simulink model "cps_base_processor_v2"  (R2012b)
settings: Solver=FixedStepDiscrete  StartTime=0.0  StopTime=8.5  FixedStep=0.005  RelTol=20e-5
model workspace (MAT data in the model file):
  vel_effective_zero = 0.0001
  pos_precision = 0.0006
  board_vpos = 0
  block_height = 0.07
libraries: simulink x4, cps_lib_v2 x3
settings Model: Creator=pmosterm  LastModifiedBy=pmosterm
settings SolverCC: ZcThreshold=2e-5  MaxConsecutiveZCs=20  EnableConcurrentExecution=on  ConcurrentTasks=on  ZeroCrossAlgorithm=Adaptive  SolverResetMethod=Robust
settings DataIOCC: SignalLoggingSaveFormat=ModelDataLogs
settings OptimizationCC: InlineParams=on  ZeroExternalMemoryAtStartup=off  ZeroInternalMemoryAtStartup=off  OptimizeModelRefInitCode=on
settings DebuggingCC: AlgebraicLoopMsg=error  UnderspecifiedInitializationDetection=Simplified  FcnCallInpInsideContextMsg=EnableAllAsWarning  BusObjectLabelMismatch=error  ModelReferenceExtraNoncontSigs=warning
settings ModelReferenceCC: ModelReferenceNumInstancesAllowed=Single
settings RTWCC: SystemTargetFile=autosar.tlc  GenCodeOnly=on  TemplateMakefile=ert_default_tmf  Description=AUTOSAR  ProcessScript=autosar_make_rtw_hook
settings CodeAppCC: IgnoreCustomStorageClasses=off
settings STFCustomTargetCC: CodeReplacementLibrary=ANSI_C  ParMdlRefBuildCompliant=on  CompOptLevelCompliant=on  IncludeMdlTerminateFcn=off  CombineOutputUpdateFcns=on  SuppressErrorStatus=on  ERTFirstTimeCompliant=on  ERTCustomFileBanners=on  SupportNonFinite=off  SupportComplex=off  SupportContinuousTime=off  SupportNonInlinedSFcns=off  AutosarCompliant=on  GRTInterface=off  SystemTargetFile=autosar.tlc
settings ERTTargetCC: CodeReplacementLibrary=ANSI_C  MultiwordLength=2048  ConcurrentExecutionCompliant=off  IncludeMdlTerminateFcn=off  SuppressErrorStatus=on  SupportNonFinite=off  SupportComplex=off  ModelStepFunctionPrototypeControlCompliant=off  CPPClassGenCompliant=off  AutosarCompliant=on  InlinedParameterPlacement=NonHierarchical  ERTCustomFileTemplate=example_file_process.tlc  ConvertIfToSwitch=off  SuppressUnreachableDefaultCases=off
settings ConfigurationSet: Description=SimMechanics 2G

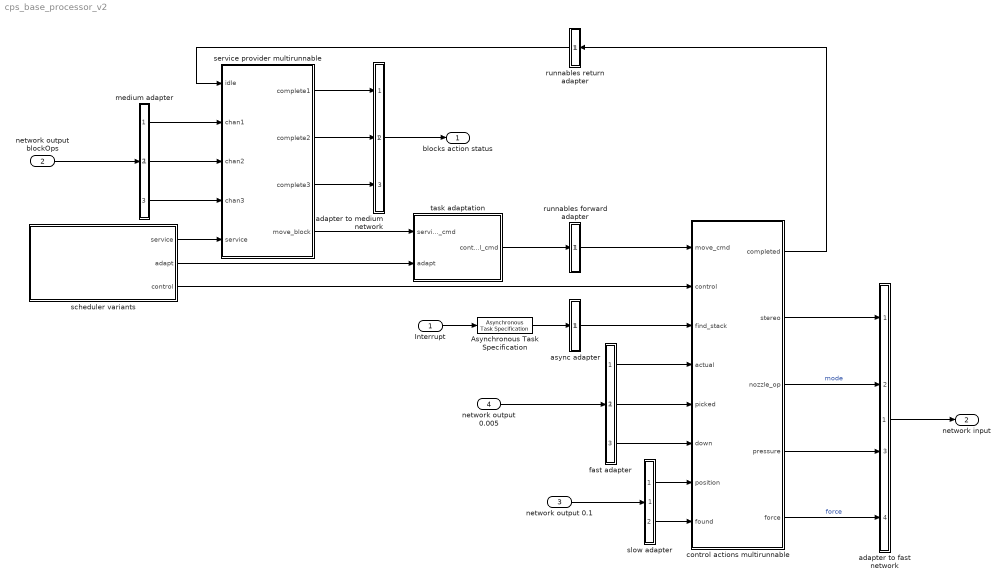
== system cps_base_processor_v2 ==
  Interrupt : Inport  OutputFunctionCall=on
  network output blockOps : Inport  Port=2  OutDataTypeStr=Bus: slBusBlockOps  PortDimensions=3  SampleTime=0.05  BusOutputAsStruct=on
  network output 0.1 : Inport  Port=3  OutDataTypeStr=Bus: slBusStereoOps  SampleTime=0.1  BusOutputAsStruct=on
  network output 0.005 : Inport  Port=4  OutDataTypeStr=Bus: slBusSliderStatus  BusOutputAsStruct=on
  Asynchronous Task Specification : AsynchronousTaskSpecification
  adapter to fast network : Subsystem
      mask Display:
      | patch([0 10 10 0], [0 0 12 0], [1 1 1]);
      | patch([0 10 0 0], [0 12 12 0], [0 0 0]);
      | 
      | plot([0 10 10 0 0], [0 0 12 12 0]);
  adapter to medium network : Subsystem
      mask Display:
      | patch([0 10 10 0], [0 0 12 0], [1 1 1]);
      | patch([0 10 0 0], [0 12 12 0], [0 0 0]);
      | 
      | plot([0 10 10 0 0], [0 0 12 12 0]);
  async adapter : Subsystem
      mask Display:
      | patch([0 10 10 0], [0 0 12 0], [0 0 0]);
      | patch([0 10 0 0], [0 12 12 0], [1 1 1]);
      | 
      | plot([0 10 10 0 0], [0 0 12 12 0]);
  control actions multirunnable : Subsystem
      mask Display:
      | patch([0 13 13 0], [0 0 11 11], [1 1 1]);
      | 
      | patch([1 7 13 1], [0 5 0 0], [0 0 0]);
      | patch([1 7 13 1], [11 6 11 11], [0 0 0]);
      | 
      | plot([7 7], [0 11]);
      | plot([0 13 13 0], [0 0 12 12]);
      | 
      | patch([14 41 41 14 14], [0 0 12 12 0], [1 1 1]);
      | plot([13 42 42 13 13], [0 0 12 12 0]);
      | 
      | text(17,6,'run()');
  fast adapter : Subsystem
      mask Display:
      | patch([0 10 10 0], [0 0 12 0], [0 0 0]);
      | patch([0 10 0 0], [0 12 12 0], [1 1 1]);
      | 
      | plot([0 10 10 0 0], [0 0 12 12 0]);
  medium adapter : Subsystem
      mask Display:
      | patch([0 10 10 0], [0 0 12 0], [0 0 0]);
      | patch([0 10 0 0], [0 12 12 0], [1 1 1]);
      | 
      | plot([0 10 10 0 0], [0 0 12 12 0]);
  runnables forward adapter : Subsystem
      mask Display:
      | patch([0 10 10 0 0], [0 0 10 10 0], [1 1 1]);
      | 
      | patch([0 5 5 0 0], [0 0 4 4 0], [0 0 0]);
      | patch([5 9 9 5 5], [5 5 9 9 5], [0 0 0]);
      | 
      | plot([0 10 10 0 0], [0 0 10 10 0]);
  runnables return adapter : Subsystem
      mask Display:
      | patch([0 10 10 0 0], [0 0 10 10 0], [1 1 1]);
      | 
      | patch([0 5 5 0 0], [0 0 4 4 0], [0 0 0]);
      | patch([5 9 9 5 5], [5 5 9 9 5], [0 0 0]);
      | 
      | plot([0 10 10 0 0], [0 0 10 10 0]);
  scheduler variants : Subsystem  Variant=on
  service provider multirunnable : Subsystem
      mask Display:
      | patch([0 13 13 0], [0 0 11 11], [1 1 1]);
      | 
      | patch([1 7 13 1], [0 5 0 0], [0 0 0]);
      | patch([1 7 13 1], [11 6 11 11], [0 0 0]);
      | 
      | plot([7 7], [0 11]);
      | plot([0 13 13 0], [0 0 12 12]);
      | 
      | patch([14 41 41 14 14], [0 0 12 12 0], [1 1 1]);
      | plot([13 42 42 13 13], [0 0 12 12 0]);
      | 
      | text(17,6,'run()');
  slow adapter : Subsystem
      mask Display:
      | patch([0 10 10 0], [0 0 12 0], [0 0 0]);
      | patch([0 10 0 0], [0 12 12 0], [1 1 1]);
      | 
      | plot([0 10 10 0 0], [0 0 12 12 0]);
  task adaptation : Subsystem
      mask Display:
      | patch([0 13 13 0], [0 0 11 11], [1 1 1]);
      | 
      | patch([1 7 13 1], [0 5 0 0], [0 0 0]);
      | patch([1 7 13 1], [11 6 11 11], [0 0 0]);
      | 
      | plot([7 7], [0 11]);
      | plot([0 13 13 0], [0 0 12 12]);
      | 
      | patch([14 41 41 14 14], [0 0 12 12 0], [1 1 1]);
      | plot([13 42 42 13 13], [0 0 12 12 0]);
      | 
      | text(17,6,'run()');
  blocks action status : Outport  SampleTime=0.05  BusOutputAsStruct=on
  network input : Outport  Port=2  OutDataTypeStr=Bus: slBusBaseOps  SampleTime=0.005  BusOutputAsStruct=on
  wires:
  scheduler variants/1(service) -> service provider multirunnable/5(service)
  scheduler variants/3(control) -> control actions multirunnable/2(control)
  network output blockOps/1 -> medium adapter/1(ops)
  medium adapter/1(R) -> service provider multirunnable/2(chan1)
  medium adapter/2(G) -> service provider multirunnable/3(chan2)
  network output 0.005/1 -> fast adapter/1(In1)
  fast adapter/1(Out1) -> control actions multirunnable/4(actual)
  fast adapter/2(Out2) -> control actions multirunnable/5(picked)
  fast adapter/3(Out3) -> control actions multirunnable/6(down)
  network output 0.1/1 -> slow adapter/1(In1)
  slow adapter/1(Out1) -> control actions multirunnable/7(position)
  slow adapter/2(Out2) -> control actions multirunnable/8(found)
  service provider multirunnable/1(complete1) -> adapter to medium network/1(R)
  service provider multirunnable/2(complete2) -> adapter to medium network/2(G)
  adapter to medium network/1(status) -> blocks action status/1
  control actions multirunnable/2(stereo) -> adapter to fast network/1(In1)
  control actions multirunnable/3(nozzle_op) -> adapter to fast network/2(In2)  "mode"
  control actions multirunnable/4(pressure) -> adapter to fast network/3(In3)
  control actions multirunnable/5(force) -> adapter to fast network/4(In4)  "force"
  adapter to fast network/1(Out1) -> network input/1
  Interrupt/1 -> Asynchronous Task Specification/1
  async adapter/1(find stack) -> control actions multirunnable/3(find_stack)
  Asynchronous Task Specification/1 -> async adapter/1(start operation)
  medium adapter/3(B) -> service provider multirunnable/4(chan3)
  service provider multirunnable/3(complete3) -> adapter to medium network/3(B)
  scheduler variants/2(adapt) -> task adaptation/2(adapt)
  service provider multirunnable/4(move_block) -> task adaptation/1(service_cmd)
  control actions multirunnable/1(completed) -> runnables return adapter/1(In1)
  runnables return adapter/1(Out1) -> service provider multirunnable/1(idle)
  task adaptation/1(control_cmd) -> runnables forward adapter/1(In1)
  runnables forward adapter/1(Out1) -> control actions multirunnable/1(move_cmd)

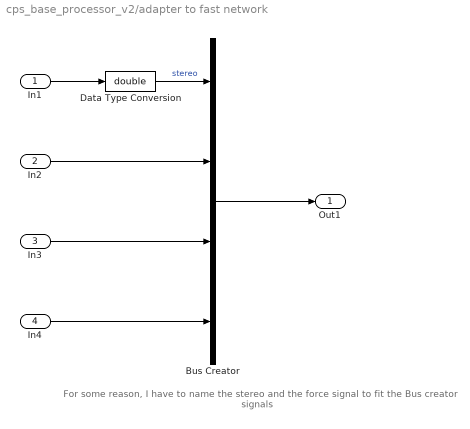
== system cps_base_processor_v2/adapter to fast network ==
  note: For some reason, I have to name
      | the stereo and the force signal
      | to fit the Bus creator signals
  In1 : Inport
  In2 : Inport  Port=2
  In3 : Inport  Port=3
  In4 : Inport  Port=4
  Bus Creator : BusCreator  Inputs='stereo','mode','pressure','force'  OutDataTypeStr=Bus: slBusBaseOps  NonVirtualBus=on
  Data Type Conversion : DataTypeConversion  OutDataTypeStr=double
  Out1 : Outport
  wires:
  Bus Creator/1 -> Out1/1
  In1/1 -> Data Type Conversion/1
  In3/1 -> Bus Creator/3
  In4/1 -> Bus Creator/4
  Data Type Conversion/1 -> Bus Creator/1  "stereo"
  In2/1 -> Bus Creator/2

== system cps_base_processor_v2/adapter to medium network ==
  R : Inport
  G : Inport  Port=2
  B : Inport  Port=3
  Mux1 : Mux  Inputs=3
  Rate Transition4 : RateTransition  Integrity=off  Deterministic=off
  status : Outport
  wires:
  Rate Transition4/1 -> status/1
  Mux1/1 -> Rate Transition4/1
  R/1 -> Mux1/1
  G/1 -> Mux1/2
  B/1 -> Mux1/3

== system cps_base_processor_v2/async adapter ==
  start operation : Inport
  Rate Transition4 : RateTransition  Integrity=off  Deterministic=off
  start finding stack : Subsystem  TreatAsAtomicUnit=on
  find stack : Outport
  wires:
  start operation/1 -> start finding stack/Trigger
  start finding stack/1(find_stack) -> Rate Transition4/1
  Rate Transition4/1 -> find stack/1

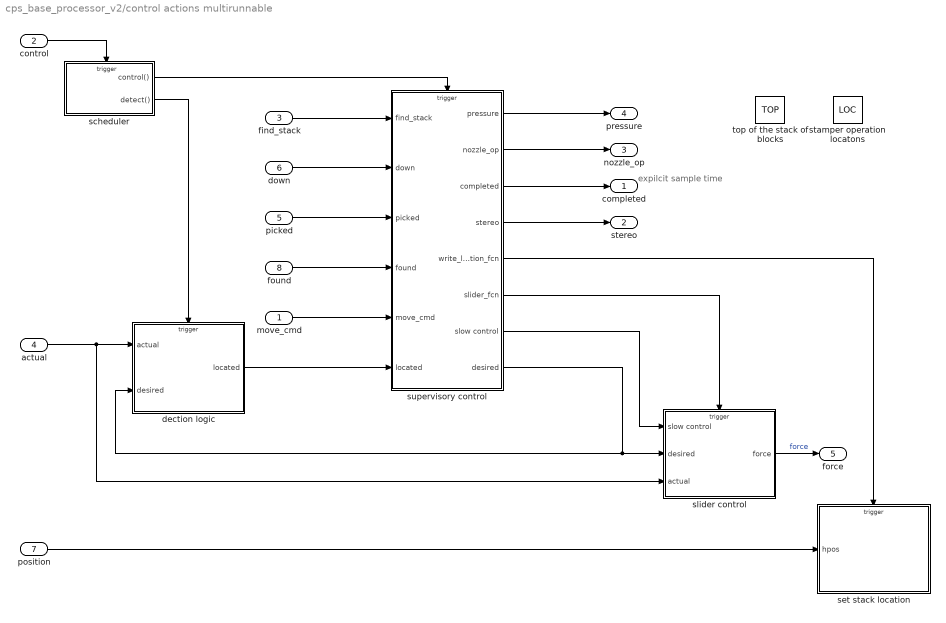
== system cps_base_processor_v2/control actions multirunnable ==
  note: expilcit sample
      | time
  move_cmd : Inport
  control : Inport  Port=2
  find_stack : Inport  Port=3
  actual : Inport  Port=4
  picked : Inport  Port=5
  down : Inport  Port=6
  position : Inport  Port=7
  found : Inport  Port=8
  dection logic : Subsystem
  scheduler : Stateflow chart  TreatAsAtomicUnit=on
  set stack location : Subsystem  TreatAsAtomicUnit=on
  slider control : Subsystem
  stamper operation locatons : DataStoreMemory  DataStoreName=LOC  WriteAfterWriteMsg=warning  InitialValue=[0.4 0.3 -0.05 -0.4 -0.6]  OutDataTypeStr=double
  supervisory control : Subsystem
  top of the stack of blocks : DataStoreMemory  DataStoreName=TOP  WriteAfterWriteMsg=warning  InitialValue=[0 0 0 3 0]  OutDataTypeStr=double
  completed : Outport
  stereo : Outport  Port=2
  nozzle_op : Outport  Port=3
  pressure : Outport  Port=4
  force : Outport  Port=5
  wires:
  position/1 -> set stack location/1(hpos)
  actual/1 -> dection logic/1(actual), slider control/3(actual)
  slider control/1(force) -> force/1  "force"
  find_stack/1 -> supervisory control/1(find_stack)
  down/1 -> supervisory control/2(down)
  picked/1 -> supervisory control/3(picked)
  found/1 -> supervisory control/4(found)
  move_cmd/1 -> supervisory control/5(move_cmd)
  dection logic/1(located) -> supervisory control/6(located)
  supervisory control/1(pressure) -> pressure/1
  supervisory control/2(nozzle_op) -> nozzle_op/1
  supervisory control/3(completed) -> completed/1
  supervisory control/6(slider_fcn) -> slider control/Trigger
  supervisory control/5(write_location_fcn) -> set stack location/Trigger
  scheduler/1(control()) -> supervisory control/Trigger
  scheduler/2(detect()) -> dection logic/Trigger
  supervisory control/4(stereo) -> stereo/1
  supervisory control/7(slow control) -> slider control/1(slow control)
  supervisory control/8(desired) -> slider control/2(desired), dection logic/2(desired)
  control/1 -> scheduler/Trigger

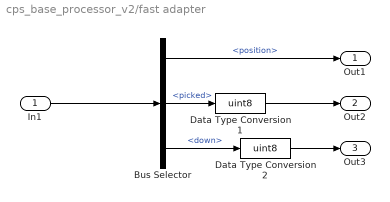
== system cps_base_processor_v2/fast adapter ==
  In1 : Inport
  Bus Selector : BusSelector  OutputSignals=position,picked,down
  Data Type Conversion1 : DataTypeConversion  OutDataTypeStr=uint8
  Data Type Conversion2 : DataTypeConversion  OutDataTypeStr=uint8
  Out1 : Outport
  Out2 : Outport  Port=2
  Out3 : Outport  Port=3
  wires:
  In1/1 -> Bus Selector/1
  Bus Selector/1 -> Out1/1  "<position>"
  Bus Selector/2 -> Data Type Conversion1/1  "<picked>"
  Bus Selector/3 -> Data Type Conversion2/1  "<down>"
  Data Type Conversion1/1 -> Out2/1
  Data Type Conversion2/1 -> Out3/1

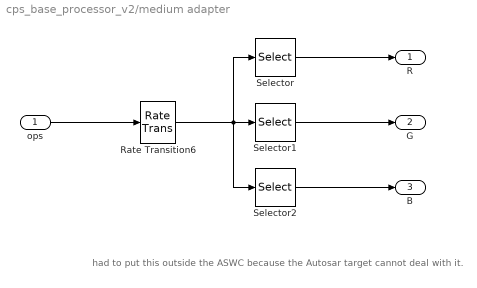
== system cps_base_processor_v2/medium adapter ==
  note: had to put this outside the ASWC
      | because the Autosar target
      | cannot deal with it.
  ops : Inport
  Rate Transition6 : RateTransition  Integrity=off  Deterministic=off
  Selector : Selector  InputPortWidth=3  IndexOptions=Index vector (dialog)  Indices=1  OutputSizes=1
  Selector1 : Selector  InputPortWidth=3  IndexOptions=Index vector (dialog)  Indices=2  OutputSizes=1
  Selector2 : Selector  InputPortWidth=3  IndexOptions=Index vector (dialog)  Indices=3  OutputSizes=1
  R : Outport
  G : Outport  Port=2
  B : Outport  Port=3
  wires:
  ops/1 -> Rate Transition6/1
  Rate Transition6/1 -> Selector2/1, Selector/1, Selector1/1
  Selector/1 -> R/1
  Selector1/1 -> G/1
  Selector2/1 -> B/1

== system cps_base_processor_v2/runnables forward adapter ==
  note: to break dependencies
      | for Autosar target
  In1 : Inport
  Rate Transition3 : RateTransition  Integrity=off  Deterministic=off
  Unit Delay : UnitDelay  SampleTime=-1
  Out1 : Outport
  wires:
  Rate Transition3/1 -> Out1/1
  In1/1 -> Unit Delay/1
  Unit Delay/1 -> Rate Transition3/1

== system cps_base_processor_v2/runnables return adapter ==
  note: to break dependencies
      | for Autosar target
      | otherwise this is only
      | necessary for the multirate
      | scheduler variant
  In1 : Inport
  Rate Transition1 : RateTransition  Integrity=off  Deterministic=off
  Unit Delay : UnitDelay  SampleTime=-1
  Out1 : Outport
  wires:
  Rate Transition1/1 -> Out1/1
  In1/1 -> Unit Delay/1
  Unit Delay/1 -> Rate Transition1/1

== system cps_base_processor_v2/scheduler variants ==
  note: 1) Only subsystems can be added as variant choices at this level
      | 2) Blocks cannot be connected at this level as connectivity is
      | automatically determined at simulation, based on the active variant
  multi rate scheduling : Subsystem  VariantObject=useMultirateVariant
  single rate conditional schaduler : Subsystem  VariantObject=noMultirateVariant
  service : Outport
  adapt : Outport  Port=2
  control : Outport  Port=3

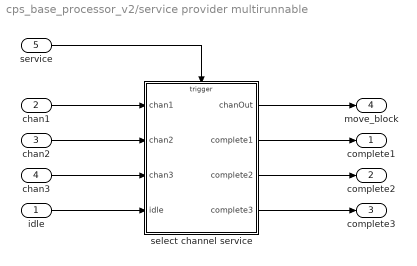
== system cps_base_processor_v2/service provider multirunnable ==
  idle : Inport
  chan1 : Inport  Port=2
  chan2 : Inport  Port=3
  chan3 : Inport  Port=4
  service : Inport  Port=5
  select channel service : Stateflow chart  TreatAsAtomicUnit=on
  complete1 : Outport
  complete2 : Outport  Port=2
  complete3 : Outport  Port=3
  move_block : Outport  Port=4
  wires:
  idle/1 -> select channel service/4(idle)
  select channel service/2(complete1) -> complete1/1
  select channel service/1(chanOut) -> move_block/1
  select channel service/3(complete2) -> complete2/1
  chan1/1 -> select channel service/1(chan1)
  chan2/1 -> select channel service/2(chan2)
  chan3/1 -> select channel service/3(chan3)
  select channel service/4(complete3) -> complete3/1
  service/1 -> select channel service/Trigger

== system cps_base_processor_v2/slow adapter ==
  In1 : Inport
  Bus Selector1 : BusSelector  OutputSignals=location,found
  Data Type Conversion3 : DataTypeConversion  OutDataTypeStr=uint16
  Rate Transition3 : RateTransition  Integrity=off  Deterministic=off
  Out1 : Outport
  Out2 : Outport  Port=2
  wires:
  In1/1 -> Rate Transition3/1
  Rate Transition3/1 -> Bus Selector1/1
  Bus Selector1/1 -> Out1/1  "<location>"
  Bus Selector1/2 -> Data Type Conversion3/1  "<found>"
  Data Type Conversion3/1 -> Out2/1

== system cps_base_processor_v2/task adaptation ==
  service_cmd : Inport
  adapt : Inport  Port=2
  location index offset : Subsystem
  control_cmd : Outport
  wires:
  service_cmd/1 -> location index offset/1(service_cmd)
  adapt/1 -> location index offset/Trigger
  location index offset/1(control_cmd) -> control_cmd/1

== system cps_base_processor_v2/async adapter/start finding stack ==
  fcn : TriggerPort  TriggerType=function-call  PortDimensions=1
  constant : Constant  SampleTime=-1
  find_stack : Outport  OutDataTypeStr=double  PortDimensions=1  OutputWhenDisabled=reset  InitialOutput=0
  wires:
  constant/1 -> find_stack/1

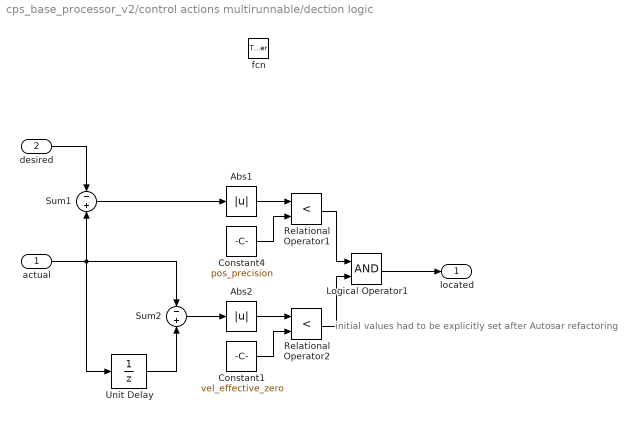
== system cps_base_processor_v2/control actions multirunnable/dection logic ==
  note: initial values had to be explicitly set
      | after Autosar refactoring
  actual : Inport
  desired : Inport  Port=2
  fcn : TriggerPort  TriggerType=function-call  PortDimensions=1
  Abs1 : Abs  ZeroCross=off
  Abs2 : Abs  ZeroCross=off
  Constant1 : Constant  Value=vel_effective_zero  OutDataTypeStr=double
  Constant4 : Constant  Value=pos_precision  OutDataTypeStr=double
  Logical Operator1 : Logic  AllPortsSameDT=off  OutDataTypeStr=boolean
  Relational Operator1 : RelationalOperator  Operator=<  OutDataTypeStr=boolean  ZeroCross=off
  Relational Operator2 : RelationalOperator  Operator=<  OutDataTypeStr=boolean  ZeroCross=off
  Sum1 : Sum  Inputs=-|+
  Sum2 : Sum  Inputs=-|+
  Unit Delay : UnitDelay  SampleTime=-1
  located : Outport  OutDataTypeStr=boolean  PortDimensions=1  InitialOutput=0
  wires:
  Constant4/1 -> Relational Operator1/2
  Sum1/1 -> Abs1/1
  Abs1/1 -> Relational Operator1/1
  actual/1 -> Sum2/1, Unit Delay/1, Sum1/2
  Relational Operator1/1 -> Logical Operator1/1
  Relational Operator2/1 -> Logical Operator1/2
  desired/1 -> Sum1/1
  Abs2/1 -> Relational Operator2/1
  Sum2/1 -> Abs2/1
  Constant1/1 -> Relational Operator2/2
  Unit Delay/1 -> Sum2/2
  Logical Operator1/1 -> located/1

== system cps_base_processor_v2/control actions multirunnable/set stack location ==
  hpos : Inport
  fcn : TriggerPort  TriggerType=function-call
  Demux : Demux  Outputs=5
  LOC = [min pos1 pos2 pos3 max] : DataStoreRead  DataStoreName=LOC
  Mux : Mux  Inputs=5
  Terminator : Terminator
  stamper locations : DataStoreWrite  DataStoreName=LOC
  wires:
  LOC = [min pos1 pos2 pos3 max]/1 -> Demux/1
  Demux/2 -> Mux/2
  Demux/3 -> Mux/3
  Demux/4 -> Terminator/1
  Demux/5 -> Mux/5
  Mux/1 -> stamper locations/1
  hpos/1 -> Mux/4
  Demux/1 -> Mux/1

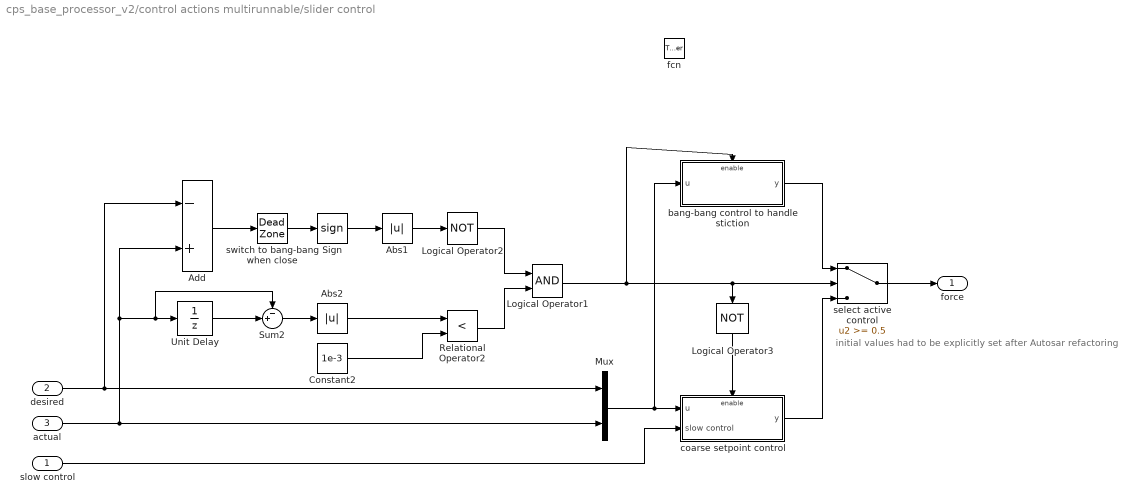
== system cps_base_processor_v2/control actions multirunnable/slider control ==
  note: initial values had to be explicitly set
      | after Autosar refactoring
  slow control : Inport  OutDataTypeStr=boolean  PortDimensions=1
  desired : Inport  Port=2  OutDataTypeStr=double  PortDimensions=1
  actual : Inport  Port=3  OutDataTypeStr=double  PortDimensions=1
  fcn : TriggerPort  TriggerType=function-call  PortDimensions=1
  Abs1 : Abs  ZeroCross=off
  Abs2 : Abs  ZeroCross=off
  Add : Sum  Inputs=-+
  Constant2 : Constant  Value=1e-3  OutDataTypeStr=double
  Logical Operator1 : Logic  AllPortsSameDT=off  OutDataTypeStr=boolean
  Logical Operator2 : Logic  Operator=NOT  AllPortsSameDT=off  OutDataTypeStr=boolean
  Logical Operator3 : Logic  Operator=NOT  AllPortsSameDT=off  OutDataTypeStr=boolean
  Mux : Mux  Inputs=2
  Relational Operator2 : RelationalOperator  Operator=<  OutDataTypeStr=boolean  ZeroCross=off
  Sign : Signum
  Sum2 : Sum  Inputs=-+|
  Unit Delay : UnitDelay  SampleTime=-1
  bang-bang control to handle stiction : Subsystem  TreatAsAtomicUnit=on
  coarse setpoint control : Subsystem  TreatAsAtomicUnit=on
  select active control : Switch  Threshold=0.5
  switch to bang-bang when close : DeadZone  LowerValue=-0.11  UpperValue=0.11  SaturateOnIntegerOverflow=on
  force : Outport  OutDataTypeStr=double  PortDimensions=1  OutputWhenDisabled=reset  InitialOutput=0
  wires:
  Mux/1 -> bang-bang control to handle stiction/1(u), coarse setpoint control/1(u)
  bang-bang control to handle stiction/1(y) -> select active control/1
  coarse setpoint control/1(y) -> select active control/3
  desired/1 -> Add/1, Mux/1
  Add/1 -> switch to bang-bang when close/1
  switch to bang-bang when close/1 -> Sign/1
  Sign/1 -> Abs1/1
  actual/1 -> Add/2, Sum2/1, Unit Delay/1, Mux/2
  Abs2/1 -> Relational Operator2/1
  Sum2/1 -> Abs2/1
  Constant2/1 -> Relational Operator2/2
  Unit Delay/1 -> Sum2/2
  Relational Operator2/1 -> Logical Operator1/2
  Abs1/1 -> Logical Operator2/1
  Logical Operator2/1 -> Logical Operator1/1
  Logical Operator3/1 -> coarse setpoint control/Enable
  Logical Operator1/1 -> select active control/2, Logical Operator3/1, bang-bang control to handle stiction/Enable
  select active control/1 -> force/1
  slow control/1 -> coarse setpoint control/2(slow control)

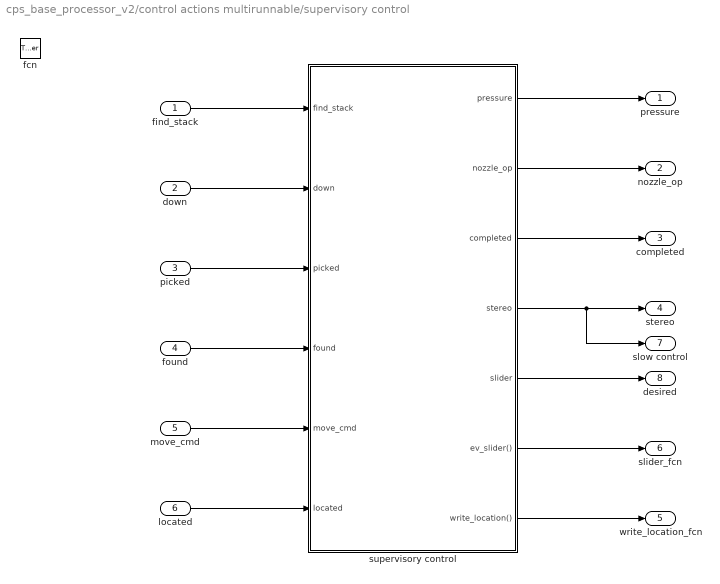
== system cps_base_processor_v2/control actions multirunnable/supervisory control ==
  find_stack : Inport
  down : Inport  Port=2
  picked : Inport  Port=3
  found : Inport  Port=4
  move_cmd : Inport  Port=5
  located : Inport  Port=6
  fcn : TriggerPort  TriggerType=function-call  PortDimensions=1
  supervisory control : Stateflow chart  TreatAsAtomicUnit=on
  pressure : Outport  InitialOutput=0
  nozzle_op : Outport  Port=2  InitialOutput=0
  completed : Outport  Port=3  InitialOutput=0
  stereo : Outport  Port=4  InitialOutput=0
  write_location_fcn : Outport  Port=5
  slider_fcn : Outport  Port=6
  slow control : Outport  Port=7  InitialOutput=0
  desired : Outport  Port=8  InitialOutput=0
  wires:
  found/1 -> supervisory control/4(found)
  move_cmd/1 -> supervisory control/5(move_cmd)
  down/1 -> supervisory control/2(down)
  supervisory control/3(completed) -> completed/1
  supervisory control/2(nozzle_op) -> nozzle_op/1
  supervisory control/6(ev_slider()) -> slider_fcn/1
  supervisory control/7(write_location()) -> write_location_fcn/1
  picked/1 -> supervisory control/3(picked)
  supervisory control/1(pressure) -> pressure/1
  find_stack/1 -> supervisory control/1(find_stack)
  located/1 -> supervisory control/6(located)
  supervisory control/4(stereo) -> stereo/1, slow control/1
  supervisory control/5(slider) -> desired/1

== system cps_base_processor_v2/scheduler variants/multi rate scheduling ==
  scheduler base modulo 10 : simulink/Ports & Subsystems/Function-Call Generator  sample_time=0.05  numberOfIterations=1
  "scheduler base modulo 10 " : simulink/Ports & Subsystems/Function-Call Generator  sample_time=0.05  numberOfIterations=1
  scheduler base rate : simulink/Ports & Subsystems/Function-Call Generator  sample_time=0.005  numberOfIterations=1
  service : Outport
  adapt : Outport  Port=2
  control : Outport  Port=3
  wires:
  scheduler base rate/1 -> control/1
  scheduler base modulo 10/1 -> service/1
  "scheduler base modulo 10 "/1 -> adapt/1

== system cps_base_processor_v2/scheduler variants/single rate conditional schaduler ==
  scheduler base rate : simulink/Ports & Subsystems/Function-Call Generator  sample_time=0.005  numberOfIterations=1
  scheduler1 : Stateflow chart  TreatAsAtomicUnit=on
  service : Outport
  adapt : Outport  Port=2
  control : Outport  Port=3
  wires:
  scheduler base rate/1 -> scheduler1/Trigger
  scheduler1/1(supervision()) -> control/1
  scheduler1/2(service()) -> service/1
  scheduler1/3(adaptation()) -> adapt/1

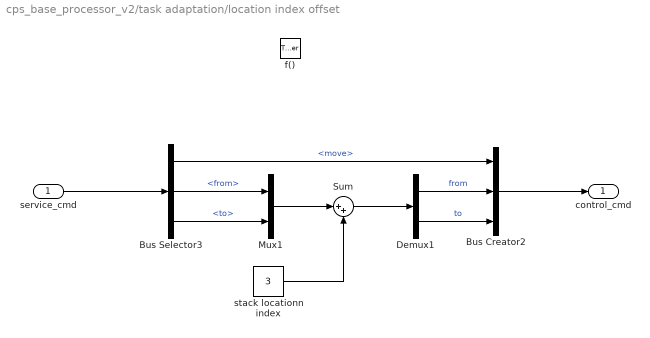
== system cps_base_processor_v2/task adaptation/location index offset ==
  service_cmd : Inport
  f() : TriggerPort  TriggerType=function-call  PortDimensions=1
  Bus Creator2 : BusCreator  Inputs='move','from','to'  OutDataTypeStr=Bus: slBusMoveBlock  NonVirtualBus=on
  Bus Selector3 : BusSelector  OutputSignals=move,from,to
  Demux1 : Demux  Outputs=2
  Mux1 : Mux  Inputs=2
  Sum : Sum  Inputs=|++
  stack locationn index : Constant  Value=3
  control_cmd : Outport  InitialOutput=0
  wires:
  Demux1/2 -> Bus Creator2/3  "to"
  Bus Selector3/3 -> Mux1/2  "<to>"
  service_cmd/1 -> Bus Selector3/1
  stack locationn index/1 -> Sum/2
  Bus Creator2/1 -> control_cmd/1
  Bus Selector3/2 -> Mux1/1  "<from>"
  Mux1/1 -> Sum/1
  Bus Selector3/1 -> Bus Creator2/1  "<move>"
  Sum/1 -> Demux1/1
  Demux1/1 -> Bus Creator2/2  "from"

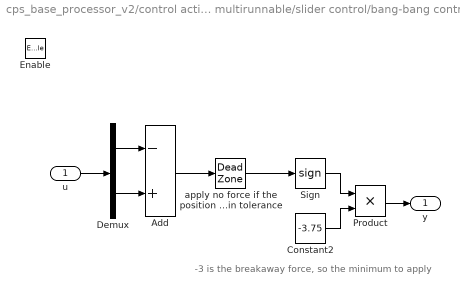
== system cps_base_processor_v2/control actions multirunnable/slider control/bang-bang control to handle stiction ==
  note: -3 is the breakaway force,
      | so the minimum to apply
  u : Inport
  Enable : EnablePort  StatesWhenEnabling=reset
  Add : Sum  Inputs=-+
  Constant2 : Constant  Value=-3.75
  Demux : Demux  Outputs=2
  Product : Product  RndMeth=Zero
  Sign : Signum
  apply no force if the position is witin tolerance : DeadZone  LowerValue=-pos_precision  UpperValue=pos_precision  SaturateOnIntegerOverflow=on
  y : Outport  OutputWhenDisabled=reset  InitialOutput=0
  wires:
  Sign/1 -> Product/1
  apply no force if the position is witin tolerance/1 -> Sign/1
  Add/1 -> apply no force if the position is witin tolerance/1
  Demux/2 -> Add/2
  Demux/1 -> Add/1
  u/1 -> Demux/1
  Product/1 -> y/1
  Constant2/1 -> Product/2

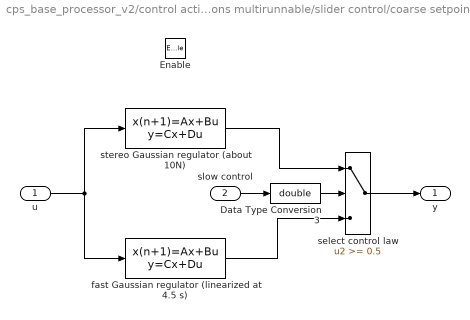
== system cps_base_processor_v2/control actions multirunnable/slider control/coarse setpoint control ==
  u : Inport
  slow control : Inport  Port=2
  Enable : EnablePort  StatesWhenEnabling=reset
  Data Type Conversion3 : DataTypeConversion  OutDataTypeStr=double
  fast Gaussian regulator (linearized at 4.5 s) : DiscreteStateSpace  A="[ 0.9940    0.0048    0.0024; -0.3823    0.9227    0.9613;  0         0    1.0000]"  B="[0.0000    0.0050;  0.0024   -0.0033;  0.0050   -0.0050]"  C="[-78.2835   -6.2453  196.8773]"  D="[0.4922   -0.6889]"  X0=[0.000000000000000 ;0.000000000000000 ;0.000000000000000 ]  SampleTime=-1  mask(DiscretizedDiscreteStateSpace){}
      mask init:
      | %zoh
  select control law : Switch  Threshold=0.5
  stereo Gaussian regulator (about 10N) : DiscreteStateSpace  A=[0.994649281526801 0.004838663977542 0.000386711916538 ;-0.134079378817680 0.940867531416425 0.153387200445988 ;0.000000000000000 0.000000000000000 1.000000000000000 ]  B=[0.000000648050558 0.005011238871482 ;0.000387363207348 -0.000703695596376 ;0.005000000000000 -0.005000000000000 ]  C=[-27.699999999999999 -2.608000000000000 31.620000000000001 ]  D=[0.000000000000000 0.000000000000000 ]  X0=[0.000000000000000 ;0.000000000000000 ;0.000000000000000 ]  SampleTime=-1  mask(DiscretizedDiscreteStateSpace){}
      mask init:
      | %zoh
  y : Outport  OutputWhenDisabled=reset  InitialOutput=0
  wires:
  u/1 -> stereo Gaussian regulator (about 10N)/1, fast Gaussian regulator (linearized at 4.5 s)/1
  slow control/1 -> Data Type Conversion3/1
  stereo Gaussian regulator (about 10N)/1 -> select control law/1
  fast Gaussian regulator (linearized at 4.5 s)/1 -> select control law/3
  select control law/1 -> y/1
  Data Type Conversion3/1 -> select control law/2

== stateflow chart cps_base_processor_v2/service provider multirunnable/select channel service ==
  state waitForInitializationSequences
  state ready
  state chan1Service
  state chan2Service
  state chan3Service
  state chan1Sync
  state chan2Sync
  state chan3Sync
  (default) -> waitForInitializationSequences
  waitForInitializationSequences -> ready : after(1,sec)
  (junction 179) -> (junction 118) : [chan1.priority > chan2.priority ...
      | && ...
      | chan1.priority > chan3.priority]
  (junction 118) -> (junction 123) [order 3]
  (junction 119) -> (junction 127) [order 2] : [chan1.priority > chan3.priority]
  (junction 127) -> (junction 162) [order 2]
  (junction 118) -> (junction 140) [order 2] : [chan3.priority > chan2.priority]
  (junction 127) -> (junction 3) [order 1]
  (junction 120) -> (junction 127) [order 3]
  (junction 118) -> (junction 3) [order 1]
  ready -> (junction 179) [order 1]
  ready -> (junction 119) [order 2] : [chan2.priority > chan1.priority ...
      | && ...
      | chan2.priority > chan3.priority]
  (junction 123) -> (junction 162) [order 2]
  (junction 119) -> (junction 140) [order 3]
  (junction 162) -> (junction 3) [order 1]
  (junction 120) -> (junction 123) [order 2] : [chan2.priority > chan1.priority]
  (junction 162) -> (junction 5) [order 2]
  (junction 140) -> (junction 162) [order 2]
  (junction 123) -> (junction 5) [order 1]
  (junction 162) -> (junction 97) [order 3]
  (junction 119) -> (junction 5) [order 1]
  (junction 55) -> ready
  ready -> (junction 177) [order 3]
  (junction 177) -> (junction 120) : [chan3.priority > chan2.priority ...
      | && ...
      | chan3.priority > chan1.priority]
  (junction 120) -> (junction 97) [order 1]
  (junction 140) -> (junction 97) [order 1]
  (junction 3) -> chan1Service : [chan1.moveBlock.move]
  (junction 5) -> chan2Service : [chan2.moveBlock.move]
  (junction 97) -> chan3Service : [chan3.moveBlock.move]
  chan1Service -> chan1Sync : [complete1]
  chan2Service -> chan2Sync : [complete2]
  chan3Service -> chan3Sync : [complete3]
  chan1Sync -> (junction 33) : after(0.5, sec)/complete1 = false;
  chan2Sync -> (junction 34) : after(0.5, sec)/complete2 = false;
  chan3Sync -> (junction 94) : after(0.5, sec)/complete3 = false;
  (junction 33) -> (junction 55)
  (junction 34) -> (junction 33)
  (junction 94) -> (junction 34)
  data: chan1 input Bus: slBusBlockOps; chan2 input Bus: slBusBlockOps; chan3 input Bus: slBusBlockOps; idle input; chanOut output Bus: slBusMoveBlock; complete1 output double; complete2 output double; complete3 output double
  events: tick input FUNCTION_CALL_EVENT

== stateflow chart cps_base_processor_v2/control actions multirunnable/supervisory control/supervisory control ==
  settings: updateMethod=DISCRETE
  state initial
  note: Variant selection for the use
      | of stereoscopic video analysis
      | based on the useStereopsis
      | variable in the MATLAB workspace
  note: The slider position control should always be active when the machine is operational,
      | otherwise (only in move_block and find_stack) a small residual velocity can accumulate
      | a large erroneous position after the control is turned off.
  state operational
    du: ev_slider;
    state idle
    note: Without ~picked, if a block is put down in a location from
        | which it should be picked up next then the picked variable
        | never has time to get reset by the slider processor control
    state find_stack
      state stereo [parallel]
        settings: executionOrder=1
        state ON
          en:
          stereo = true;
        state OFF
          en:
          stereo = false;
        (default) -> ON
        ON -> OFF : [found]/stack_found = true; write_location;
    state move_block
      state pressure [parallel]
        settings: executionOrder=2
        state initial
          en:
          pressure = 10;
        state start
          en:
          pressure = 500;
        (default) -> operational.move_block.pressure.initial
        start -> operational.move_block.pressure.initial : [in(move.place) && down]
        operational.move_block.pressure.initial -> start : [in(move.pick)]
      state move [parallel]
        settings: executionOrder=1
        state move2pos
          en:
          slider = LOC[from];
          nozzle_op.mode = neutral;
        state pick
          en:
          nozzle_op.TOP = TOP[from];
          nozzle_op.mode = NozzleOps.action;
        state position
          en:
          slider = LOC[to];
          nozzle_op.mode = NozzleOps.motion;
        state place
          en:
          nozzle_op.TOP = TOP[to];
          nozzle_op.mode = NozzleOps.action;
          ex:
          nozzle_op.mode = neutral;
        (default) -> move2pos
        move2pos -> pick : [located]
        pick -> position : [picked]/TOP[from]--;
        position -> place : [located]/TOP[to]++;
    state sync
    (default) -> idle
    find_stack -> idle : [located]
    idle -> (junction 61)
    sync -> idle : [move_cmd.move == 0]
    (junction 61) -> (junction 66) [order 1] : [find_stack && ~stack_found]/
        | slider = LOC[4];
    (junction 61) -> (junction 159) [order 2] : [stack_found && move_cmd.move && ~picked]/
        | from = move_cmd.from; to = move_cmd.to; completed = false;
    (junction 66) -> find_stack
    (junction 159) -> move_block
    place -> sync : [picked]/
        | completed = true;
  (default) -> initial : /pressure = 0;completed = false; stack_found = false;
  initial -> (junction 161)
  (junction 161) -> (junction 162) [order 1]
  (junction 161) -> (junction 165) [order 2]
  (junction 162) -> (junction 198) : [useStereopsis]/
      | stack_found = false;
      | stereo = true;
  (junction 165) -> (junction 199) : [~useStereopsis]/
      | stack_found = true;
      | stereo = false;
  (junction 198) -> (junction 197)
  (junction 199) -> (junction 197)
  (junction 197) -> operational
  data: find_stack input double; down input uint8 size=1 =0.1; picked input; found input; LOC data_store_memory size=5; move_cmd input Bus: slBusMoveBlock; located input; pressure output double; nozzle_op output Bus: slBusNozzleOps; TOP data_store_memory; from local double; to local double; completed output double; stereo output boolean =true; slider output double; stack_found local double; useStereopsis local double =useStereopsis
  events: ev_slider output FUNCTION_CALL_EVENT; write_location output FUNCTION_CALL_EVENT

== stateflow chart cps_base_processor_v2/control actions multirunnable/scheduler ==
  state scheduler
    en: detect; control;
    du: detect; control;
  (default) -> scheduler
  events: control output FUNCTION_CALL_EVENT; detect output FUNCTION_CALL_EVENT; tick input FUNCTION_CALL_EVENT

== stateflow chart cps_base_processor_v2/scheduler variants/single rate conditional schaduler/scheduler1 ==
  state scheduler
    state OneTick [parallel]
      entry: supervision;
      on every(1,tick):
      supervision;
      settings: executionOrder=2
    state TenTick [parallel]
      entry: service; adaptation;
      on every(10,tick):
      service; adaptation;
      settings: executionOrder=1
  (default) -> scheduler
  events: supervision output FUNCTION_CALL_EVENT; service output FUNCTION_CALL_EVENT; adaptation output FUNCTION_CALL_EVENT; tick input FUNCTION_CALL_EVENT
